simulink model "buck_converter_CPM_open_loop_simscape"  (R2016a)
settings: Solver=ode23tb  StartTime=0.0  StopTime=1e-3  MaxStep=1e-7  RelTol=1e-7
values from neighbouring files (symbols this model uses):
  C = 200e-6    (= 0.0002)    [buck_converter_CPM_open_loop_simscape_parameters.m]
  Dmax = 0.9    [buck_converter_CPM_open_loop_simscape_parameters.m]
  Dmin = 0    [buck_converter_CPM_open_loop_simscape_parameters.m]
  fs = 1e6    (= 1000000)    [buck_converter_CPM_open_loop_simscape_parameters.m]
  iLmax = 5    [buck_converter_CPM_open_loop_simscape_parameters.m]
  L = 1e-6    (= 1e-06)    [buck_converter_CPM_open_loop_simscape_parameters.m]
  Resr = 0.8e-3    (= 0.0008)    [buck_converter_CPM_open_loop_simscape_parameters.m]
  Rin = 10e6    (= 10000000)    [buck_converter_CPM_open_loop_simscape_parameters.m]
  RL = 15e-3    (= 0.015)    [buck_converter_CPM_open_loop_simscape_parameters.m]
  Rload = 0.4    [buck_converter_CPM_open_loop_simscape_parameters.m]
  Rs = 0.3    [buck_converter_CPM_open_loop_simscape_parameters.m]
  Vg = 5    [buck_converter_CPM_open_loop_simscape_parameters.m]
libraries: powerlib x22, simulink_extras x1
settings Model: Creator=Gorkem  LastModifiedBy=Gorkem
settings SolverCC: AlgebraicLoopSolver=LineSearch
settings DebuggingCC: MaxConsecutiveZCsMsg=none
settings GRTTargetCC: GeneratePreprocessorConditionals=Use local settings

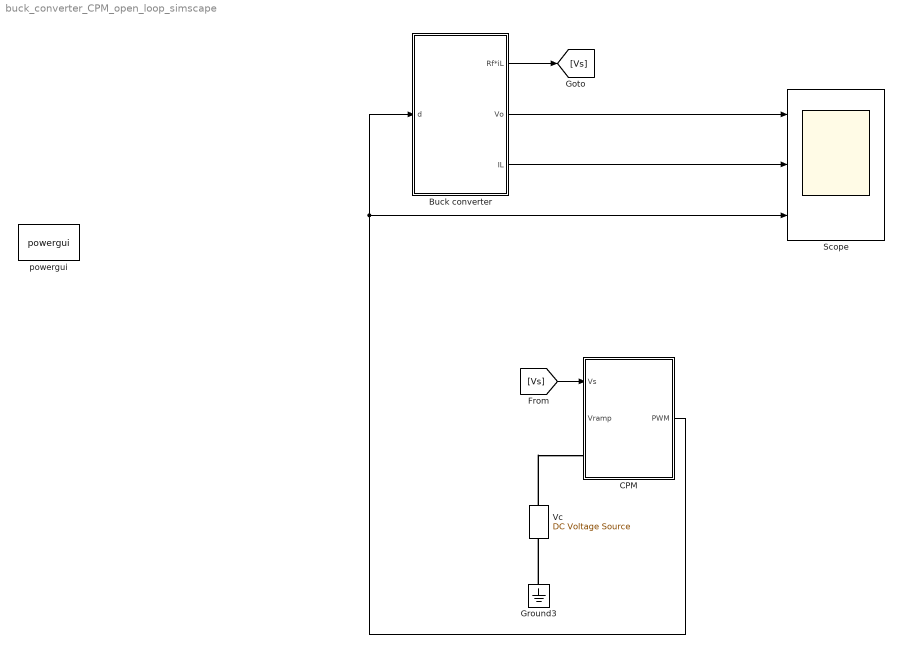
== system buck_converter_CPM_open_loop_simscape ==
  Buck converter : Subsystem
  CPM : Subsystem
  Ground3 : powerlib/Elements/Ground  LConnTagsString=a
  Scope : Scope  NumInputPorts=3
  Vc : powerlib/Electrical Sources/DC Voltage Source  Amplitude=Rs*iLmax  Measurements=None
  powergui : powerlib/powergui  Priority=1  SimulationMode=Continuous  SolverType=Tustin/Backward Euler (TBE)  SampleTime=1e-7  frequency=60  SPID=off  DisableSnubberDevices=off  DisableRonSwitches=off  DisableVfSwitches=off  SwTol=0  DisplayEquations=off  Interpol=off  ExternalGateDelay=off  methode=off  Ts=10  FunctionMessages=off  echomessages=off  HookPort=off  EnableUseOfTLC=off  x0status=blocks  frequencyindice=0  Pbase=100e6  ErrMax=1e-4  Iterations=50  UnitsV=kV  UnitsW=MW  buscounter=0  RestoreLinks=warning  ResistiveCurrentMeasurement=off  Frange=[0:2:500]  Ylog=off  Xlog=on  ShowGrid=off  save=off  variable=ZData  structure=0  ZoomFFT=off  StartTime=0.0  cycles=1  DisplayStyle=1  fundamental=60  FreqAxis=off  MaxFrequency=1000  frequencyindicesteady=1  RmsSteady=1  display=off
  wires:
  CPM/1(PWM) -> Scope/3, Buck converter/1(d)
  Buck converter/2(Vo) -> Scope/1
  Buck converter/3(IL) -> Scope/2
  Buck converter/1(Rf*iL) -> [Vs]
  [Vs] -> CPM/1(Vs)
  connections:
  Ground3/LConn1 -- Vc/LConn1
  Vc/RConn1 -- CPM/LConn1

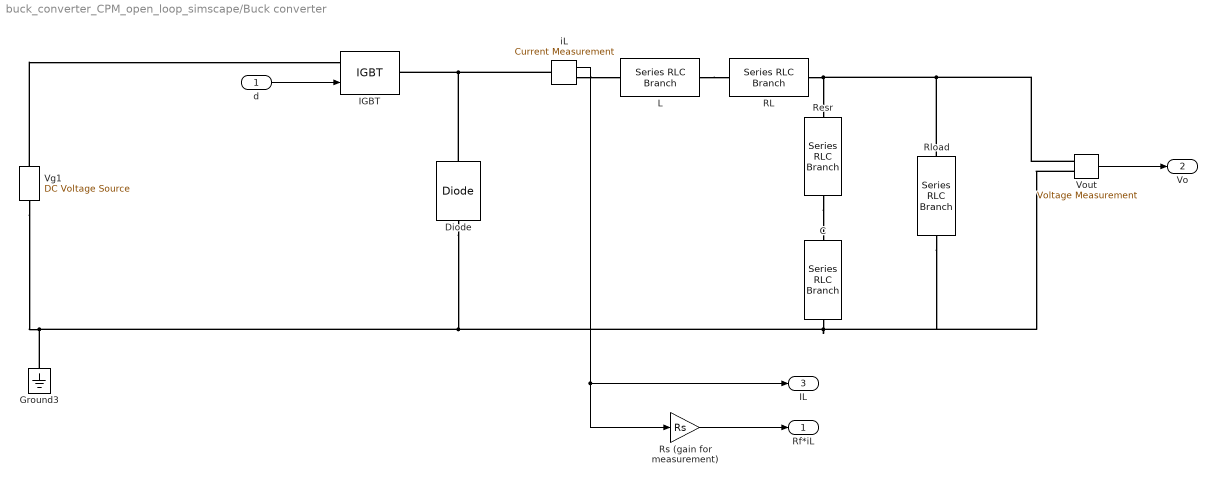
== system buck_converter_CPM_open_loop_simscape/Buck converter ==
  d : Inport
  C : powerlib/Elements/Series RLC Branch  LConnTagsString=__new0  RConnTagsString=__new0  BranchType=C  Resistance=1  Inductance=L  SetiL0=off  InitialCurrent=0  Capacitance=C  Setx0=off  InitialVoltage=0  Measurements=None
  Diode : powerlib/Power Electronics/Diode  Ron=0.001  Lon=0  Vf=0.6  IC=0  UseSnubber=off  Rs=500  Cs=250e-9  Measurements=off
  Ground3 : powerlib/Elements/Ground  LConnTagsString=a
  IGBT : powerlib/Power Electronics/IGBT  Ron=0.001  Lon=0  Vf=0.5  Tf=1e-6  Tt=2e-6  IC=0  Rs=1e5  Cs=inf  Measurements=off
  L : powerlib/Elements/Series RLC Branch  LConnTagsString=__new0  RConnTagsString=__new0  BranchType=L  Resistance=1  Inductance=L  SetiL0=off  InitialCurrent=0  Capacitance=1e-6  Setx0=off  InitialVoltage=0  Measurements=None
  RL : powerlib/Elements/Series RLC Branch  LConnTagsString=__new0  RConnTagsString=__new0  BranchType=R  Resistance=RL  Inductance=L  SetiL0=off  InitialCurrent=0  Capacitance=C  Setx0=off  InitialVoltage=0  Measurements=None
  Resr : powerlib/Elements/Series RLC Branch  LConnTagsString=__new0  RConnTagsString=__new0  BranchType=R  Resistance=Resr  Inductance=L  SetiL0=off  InitialCurrent=0  Capacitance=C  Setx0=off  InitialVoltage=0  Measurements=None
  "Rload " : powerlib/Elements/Series RLC Branch  LConnTagsString=__new0  RConnTagsString=__new0  BranchType=R  Resistance=Rload  Inductance=L  SetiL0=off  InitialCurrent=0  Capacitance=C  Setx0=off  InitialVoltage=0  Measurements=None
  Rs (gain for measurement) : Gain  Gain=Rs
  Vg1 : powerlib/Electrical Sources/DC Voltage Source  Amplitude=Vg  Measurements=None
  Vout : powerlib/Measurements/Voltage Measurement  PhasorSimulation=off  OutputType=Complex  PSBequivalent=0
  iL : powerlib/Measurements/Current Measurement  PhasorSimulation=off  OutputType=Complex  PSBequivalent=0
  Rf*iL : Outport
  Vo : Outport  Port=2
  IL : Outport  Port=3
  wires:
  Rs (gain for measurement)/1 -> Rf*iL/1
  iL/1 -> IL/1, Rs (gain for measurement)/1
  Vout/1 -> Vo/1
  d/1 -> IGBT/1
  connections:
  Vg1/LConn1 -- Diode/LConn1 -- "Rload "/RConn1 -- Vout/LConn2 -- C/RConn1 -- Ground3/LConn1
  Diode/RConn1 -- iL/LConn1 -- IGBT/RConn1
  "Rload "/LConn1 -- Vout/LConn1 -- RL/RConn1 -- Resr/LConn1
  Vg1/RConn1 -- IGBT/LConn1
  L/RConn1 -- RL/LConn1
  iL/RConn1 -- L/LConn1
  Resr/RConn1 -- C/LConn1

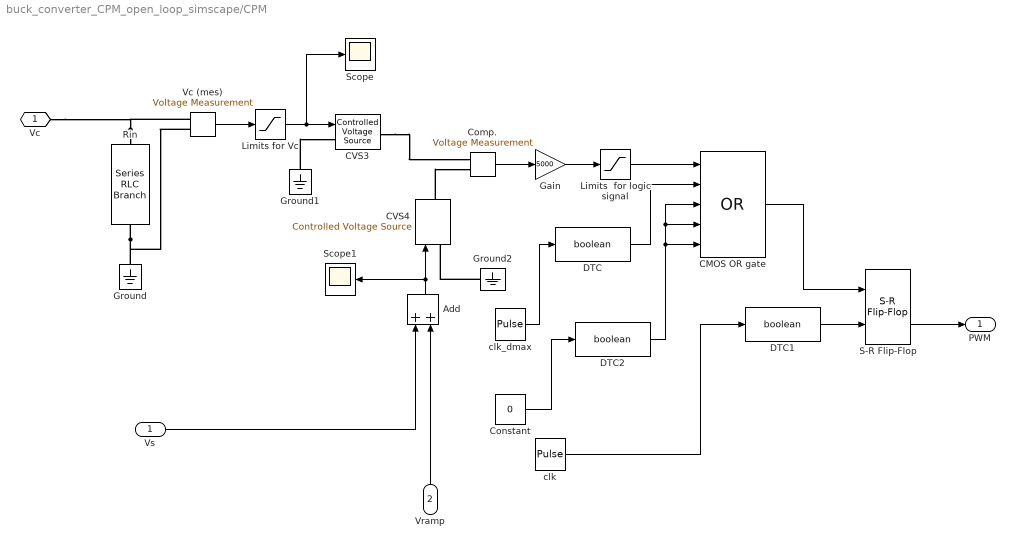
== system buck_converter_CPM_open_loop_simscape/CPM ==
  Vs : Inport
  Vramp : Inport  Port=2
  Add : Sum
  CMOS OR gate : Logic  Operator=OR  Inputs=5  AllPortsSameDT=off  OutDataTypeStr=boolean
  CVS3 : powerlib/Electrical Sources/Controlled Voltage Source  Initialize=off  Source_Type=AC  Amplitude=0  Phase=0  Frequency=0  Measurements=Voltage
  CVS4 : powerlib/Electrical Sources/Controlled Voltage Source  Initialize=off  Source_Type=AC  Amplitude=0  Phase=0  Frequency=0  Measurements=Voltage
  Comp. : powerlib/Measurements/Voltage Measurement  PhasorSimulation=off  OutputType=Complex  PSBequivalent=0
  Constant : Constant  Value=0
  DTC : DataTypeConversion  OutDataTypeStr=boolean  SaturateOnIntegerOverflow=on  LockScale=on
  DTC1 : DataTypeConversion  OutDataTypeStr=boolean  SaturateOnIntegerOverflow=on  LockScale=on
  DTC2 : DataTypeConversion  OutDataTypeStr=boolean  SaturateOnIntegerOverflow=on  LockScale=on
  Gain : Gain  Gain=5000
  Ground : powerlib/Elements/Ground  LConnTagsString=a
  Ground1 : powerlib/Elements/Ground  LConnTagsString=a
  Ground2 : powerlib/Elements/Ground  LConnTagsString=a
  Limits for Vc : Saturate  UpperLimit=5  LowerLimit=0
  "Limits  for logic signal " : Saturate  UpperLimit=1  LowerLimit=0
  Rin : powerlib/Elements/Series RLC Branch  LConnTagsString=__new0  RConnTagsString=__new0  BranchType=R  Resistance=Rin  Inductance=1e-3  SetiL0=off  InitialCurrent=0  Capacitance=1e-6  Setx0=off  InitialVoltage=0  Measurements=None
  S-R Flip-Flop : simulink_extras/Flip Flops/S-R Flip-Flop  initial_condition=0
  Scope : Scope
  Scope1 : Scope
  Vc (mes) : powerlib/Measurements/Voltage Measurement  PhasorSimulation=off  OutputType=Complex  PSBequivalent=0
  clk : DiscretePulseGenerator  PulseType=Time based  Amplitude=5  Period=1/fs  PulseWidth=(Dmin+1e-10)*100
  clk_dmax : DiscretePulseGenerator  PulseType=Time based  Amplitude=5  Period=1/fs  PulseWidth=(1-Dmax)*100  PhaseDelay=Dmax/fs
  Vc : PMIOPort  Port=1  Side=Left
  PWM : Outport
  wires:
  Vs/1 -> Add/1
  Add/1 -> CVS4/1, Scope1/1
  Limits for Vc/1 -> Scope/1, CVS3/1
  Vramp/1 -> Add/2
  Vc (mes)/1 -> Limits for Vc/1
  Comp./1 -> Gain/1
  Gain/1 -> "Limits  for logic signal "/1
  S-R Flip-Flop/2 -> PWM/1
  CMOS OR gate/1 -> S-R Flip-Flop/1
  clk_dmax/1 -> DTC/1
  DTC/1 -> CMOS OR gate/2
  DTC1/1 -> S-R Flip-Flop/2
  clk/1 -> DTC1/1
  Constant/1 -> DTC2/1
  DTC2/1 -> CMOS OR gate/5, CMOS OR gate/4, CMOS OR gate/3
  "Limits  for logic signal "/1 -> CMOS OR gate/1
  connections:
  Rin/RConn1 -- Ground/LConn1 -- Vc (mes)/LConn2
  Rin/LConn1 -- Vc (mes)/LConn1 -- Vc/RConn1
  CVS4/RConn1 -- Comp./LConn1
  Ground2/LConn1 -- CVS4/LConn1
  Ground1/LConn1 -- CVS3/LConn1
  CVS3/RConn1 -- Comp./LConn2
